simulink library "Lib_EMTAT"  (R2021b)
settings: Solver=VariableStepAuto  StartTime=0.0  StopTime=10.0  RelTol=1e-3
undefined symbols (not defined in the file or in its folder): A_M, B_M, Cj, component_degradation_input, Cs, E0_M, f_sw, K_M, MWS, Q_M, Q_rr, r_c, r_D, R_M, Rj, Ru, SNR_DX_M, SNR_IC_M, SNR_Mn_M, SNR_Mx_M, SOC_Init_M, u_ce0, u_D0
libraries: $bdroot x82, simulink x23, Lib_Dyn_StateSpace_EMTAT x3, PB_Library_Master_Working x1
(part 7 of 7)

== system Lib_EMTAT/Components/Power Flow/Three Phase Electric Machine (Source)/Open Circuit Failure - Line-Neutral Voltage ==
  Failed? : Inport
  V_LN_rms : Inport  Port=2
  Constant : Constant  Value=0
  IsInf : RelationalOperator  Operator=isInf  OutDataTypeStr=boolean  RndMeth=Simplest
  IsNaN : RelationalOperator  Operator=isNaN  OutDataTypeStr=boolean  RndMeth=Simplest
  Logical Operator : Logic  Operator=OR  Inputs=3  AllPortsSameDT=off  OutDataTypeStr=boolean
  Switch : Switch  Criteria=u2 > Threshold
  "V_LN_rms " : Outport
  wires:
  IsInf/1 -> Logical Operator/3
  IsNaN/1 -> Logical Operator/2
  Logical Operator/1 -> Switch/2
  Switch/1 -> "V_LN_rms "/1
  V_LN_rms/1 -> Switch/3, IsInf/1, IsNaN/1
  Constant/1 -> Switch/1
  Failed?/1 -> Logical Operator/1

== system Lib_EMTAT/Components/Power Flow/Three Phase Electric Machine (Source)/Open Circuit// Degradation Failure ==
  Eff : Inport
  DegFail? : Inport  Port=2
  OCFail? : Inport  Port=3
  Deg : Inport  Port=4
  Constant : Constant  Value=0
  Constant1 : Constant
  Divide : Product  Inputs=**
  "If degradation failure, penalize Eff." : Switch  Criteria=u2 > Threshold
  "If open circuit failure, set Eff = 0." : Switch  Criteria=u2 > Threshold
  Sum : Sum  Inputs=+-|
  "Eff " : Outport
  wires:
  Sum/1 -> Divide/1
  Constant1/1 -> Sum/1
  Constant/1 -> "If open circuit failure, set Eff = 0."/1
  OCFail?/1 -> "If open circuit failure, set Eff = 0."/2
  "If open circuit failure, set Eff = 0."/1 -> "Eff "/1
  Deg/1 -> Sum/2
  Divide/1 -> "If degradation failure, penalize Eff."/1
  Eff/1 -> "If degradation failure, penalize Eff."/3, Divide/2
  "If degradation failure, penalize Eff."/1 -> "If open circuit failure, set Eff = 0."/3
  DegFail?/1 -> "If degradation failure, penalize Eff."/2

== system Lib_EMTAT/Numerical Methods/Newton Raphson Solver/NR Update/Bounding ==
  note: Throw warning if solver independents reach independent limits.
  note: Throw error if initial condition is zero. This will disrupt normalization within solver.
  note: Throw error if initial conditions set in mask are not within independent limits set in mask.
  x(n+1)raw : Inport
  HitLimits : Subsystem
  ICsOutsideLimit : Subsystem
  Initial Conditions : Constant  Value=NR_IC_M
  Logical Operator{,1..3} (4 alike) : Logic  Operator=OR  AllPortsSameDT=off  OutDataTypeStr=boolean
  Memory : Memory  InheritSampleTime=on
  Memory1 : Memory  InheritSampleTime=on
  MinMax : MinMax  Inputs=2
  MinMax1 : MinMax  Function=max  Inputs=2
  Relational Operator : RelationalOperator  Operator===  OutDataTypeStr=boolean  RndMeth=Nearest
  Relational Operator1 : RelationalOperator  Operator===  OutDataTypeStr=boolean  RndMeth=Nearest
  Relational Operator2 : RelationalOperator  OutDataTypeStr=boolean  RndMeth=Nearest
  Relational Operator3 : RelationalOperator  Operator=<=  OutDataTypeStr=boolean  RndMeth=Nearest
  Relational Operator4 : RelationalOperator  Operator=isNaN  OutDataTypeStr=boolean  RndMeth=Nearest
  ZeroIC : Subsystem
  xBottom : Constant  Value=NR_Mn_Lim_M
  xTop : Constant  Value=NR_Mx_Lim_M
  x(n+1)Lim : Outport
  wires:
  Relational Operator4/1 -> ZeroIC/Enable
  [BotLim] -> Relational Operator3/2
  Relational Operator2/1 -> Logical Operator2/1
  Memory1/1 -> Logical Operator3/2
  Relational Operator3/1 -> Logical Operator2/2
  Logical Operator2/1 -> Logical Operator3/1
  [TopLim] -> Relational Operator2/2
  Initial Conditions/1 -> Relational Operator3/1, Relational Operator2/1, Relational Operator4/1
  Logical Operator3/1 -> Memory1/1, ICsOutsideLimit/Enable
  Logical Operator1/1 -> Memory/1, HitLimits/Enable
  Memory/1 -> Logical Operator1/2
  [HitBtm] -> Logical Operator/2
  Logical Operator/1 -> Logical Operator1/1
  [HitTop] -> Logical Operator/1
  Relational Operator/1 -> [HitTop]
  Relational Operator1/1 -> [HitBtm]
  MinMax/1 -> x(n+1)Lim/1, Relational Operator/2, Relational Operator1/1
  MinMax1/1 -> MinMax/2
  xTop/1 -> MinMax/1, Relational Operator/1, [TopLim]
  x(n+1)raw/1 -> MinMax1/1
  xBottom/1 -> Relational Operator1/2, MinMax1/2, [BotLim]

== system Lib_EMTAT/Numerical Methods/Newton Raphson Solver/NR Update/MatrixMult ==
  f(x(n)) : Inport
  inv(f'(x(n))) : Inport  Port=2
  Product : Product  Multiplication=Matrix(*)  RndMeth=Zero
  DTS : Outport
  wires:
  inv(f'(x(n)))/1 -> Product/1
  f(x(n))/1 -> Product/2
  Product/1 -> DTS/1

== system Lib_EMTAT/Numerical Methods/Newton Raphson Solver/NR Update/dxLimit1 ==
  dx : Inport
  f(x(n)) : Inport  Port=2
  Abs1 : Abs
  Constant : Constant  Value=0.5
  Constant1 : Constant  Value=-1
  Memory : Memory  InheritSampleTime=on
  MinMax : MinMax  Inputs=2
  MinMax1 : MinMax  Function=max  Inputs=2
  Product1 : Product  Inputs=3  RndMeth=Zero
  Product2 : Product  RndMeth=Zero
  Sum : Sum  Inputs=|++
  Threshold : Constant  Value=NR_dx_Lim_M/100
  dx_limited : Outport
  wires:
  MinMax1/1 -> dx_limited/1
  Constant1/1 -> Product2/1
  Product2/1 -> MinMax1/1
  MinMax/1 -> MinMax1/2
  dx/1 -> MinMax/2
  Abs1/1 -> MinMax/1, Product2/2
  Product1/1 -> Abs1/1
  Threshold/1 -> Product1/1
  f(x(n))/1 -> Memory/1, Sum/2
  Constant/1 -> Product1/2
  Memory/1 -> Sum/1
  Sum/1 -> Product1/3

== system Lib_EMTAT/Solvers/Iterative NR Solver w JacobianCalc/NRwCond/Iteration Conditions ==
  f(x) : Inport
  Abs : Abs
  Constant1 : Constant  Value=Cond_Limits_M
  Constant2 : Constant  Value=0
  Relational Operator : RelationalOperator  Operator=>  OutDataTypeStr=boolean  RndMeth=Nearest
  Relational Operator1 : RelationalOperator  Operator=>  OutDataTypeStr=boolean  RndMeth=Nearest
  Sum of Elements : Sum  Inputs=+
  Condition : Outport
  wires:
  Relational Operator1/1 -> Condition/1
  Sum of Elements/1 -> Relational Operator1/1
  Constant2/1 -> Relational Operator1/2
  Relational Operator/1 -> Sum of Elements/1
  f(x)/1 -> Abs/1
  Constant1/1 -> Relational Operator/2
  Abs/1 -> Relational Operator/1

== system Lib_EMTAT/Solvers/SS NR Solver w JacobianCalc /JacCalc w Reset/JC_Reset counter ==
  Reset Counter : Inport
  Count Condition : Inport  Port=2
  Constant1 : Constant  Value=SJacobianAttempts_M
  Data Type Conversion : DataTypeConversion
  Data Type Conversion1 : DataTypeConversion
  Logical Operator : Logic  Operator=NOT  AllPortsSameDT=off  OutDataTypeStr=boolean
  Product : Product  RndMeth=Zero
  Relational Operator : RelationalOperator  Operator===  OutDataTypeStr=boolean  RndMeth=Nearest
  Sum : Sum  Inputs=|++
  Unit Delay : UnitDelay  SampleTime=-1  HasFrameUpgradeWarning=on
  Unit Delay1 : UnitDelay  SampleTime=-1  HasFrameUpgradeWarning=on
  Unit Delay2 : UnitDelay  SampleTime=-1  HasFrameUpgradeWarning=on
  JC_Reset : Outport
  wires:
  Constant1/1 -> Relational Operator/1
  Relational Operator/1 -> JC_Reset/1
  Product/1 -> Sum/2
  Reset Counter/1 -> Unit Delay1/1
  Unit Delay/1 -> Product/2
  Data Type Conversion/1 -> Product/1
  Data Type Conversion1/1 -> Sum/1
  Unit Delay1/1 -> Logical Operator/1
  Logical Operator/1 -> Data Type Conversion/1
  Count Condition/1 -> Unit Delay2/1
  Unit Delay2/1 -> Data Type Conversion1/1
  Sum/1 -> Unit Delay/1, Relational Operator/2

== system Lib_EMTAT/Solvers/SS NR Solver w JacobianCalc /NewRaph w Cond/conditions ==
  f(x) : Inport
  Abs : Abs
  Constant2 : Constant  Value=Cond_Limits_M
  Constant3 : Constant  Value=0
  Relational Operator1 : RelationalOperator  Operator=>  OutDataTypeStr=boolean  RndMeth=Nearest
  Relational Operator2 : RelationalOperator  Operator=>  OutDataTypeStr=boolean  RndMeth=Nearest
  Sum of Elements : Sum  Inputs=+
  Condition : Outport
  wires:
  Constant2/1 -> Relational Operator1/2
  Relational Operator1/1 -> Sum of Elements/1
  Constant3/1 -> Relational Operator2/2
  Abs/1 -> Relational Operator1/1
  Sum of Elements/1 -> Relational Operator2/1
  f(x)/1 -> Abs/1
  Relational Operator2/1 -> Condition/1

== system Lib_EMTAT/Components/Physics-Based/Boost Converter/DC - DC Converter/ Dynamic State ==
  note: On Cycle
  note: Off Cycle
  note: the aDF must decrease L_M
  note: the aDF must decrease L_M
  x : Inport
  u : Inport  Port=2
  d : Inport  Port=3
  Action Port : ActionPort
  Constant : Constant
  Product{,1..3} (4 alike) : Product
  "State Space Model A1, B1, C1, D1" : Lib_Dyn_StateSpace_EMTAT/State Space Model  A_M=[0, 0; 0, -(Ron_M+RL_M)/L_M]  B_M=[0, -1/C_M; 1/L_M, 0]  C_M="[1,  0]"  D_M=[0, RC_M]
  "State Space Model A2, B2, C2, D2" : Subsystem  mask(State Space Model){A_M=[0, 1/C_M; -1/L_M, -(Ron_M+RC_M+RL_M)/L_M], B_M=[0, -1/C_M; 1/L_M, RC_M/L_M], C_M=[1,  RC_M], D_M=[0, -RC_M]}
      mask prompts: A_M "A_M - "A" Matrix"; B_M "B_M - "B" Matrix"; C_M "C_M - "C" Matrix"; D_M "D_M - "D" Matrix"
      mask help:
      | This block represents a state space model that can be placed within an interative subsytem (i.e. the Newton-Raphson solver).
      | The states, x, and inputs, u must be fed into the block. The outputs, y, and state derivatives, x_dot are computed
      | via the standard state space equations. Note that the integrator that computes the states by integrating
      | the state derivatives should be placed outside of the iterative subsystem so that multiple integration steps do not
      | occur per each timestep.
      |
      | Initial conditions must be specified in the integrator blocks, and ABCD matrices specified as block mask parameters.
      mask Display:
      | fprintf('x_dot = Ax+Bu\ny = Cx+Du')
      | port_label('input',1,'x')
      | port_label('input',2,'u')
      | port_label('output',1,'x_dot')
      | port_label('output',2,'y')
  Sum : Sum  Inputs=++|
  Sum1 : Sum  Inputs=++|
  Sum2 : Sum  Inputs=+-
  xdot : Outport  VectorParamsAs1DForOutWhenUnconnected=off
  VB : Outport  Port=2  VectorParamsAs1DForOutWhenUnconnected=off
  wires:
  "State Space Model A1, B1, C1, D1"/1 -> Product/1
  d/1 -> [d]
  Sum2/1 -> Product2/2, Product3/2
  Constant/1 -> Sum2/1
  [x] -> "State Space Model A1, B1, C1, D1"/1
  "State Space Model A1, B1, C1, D1"/2 -> Product1/1
  [u] -> "State Space Model A1, B1, C1, D1"/2
  [d] -> Product1/2, Product/2
  [d] -> Sum2/2
  u/1 -> [u]
  [x] -> "State Space Model A2, B2, C2, D2"/1(x)
  [u] -> "State Space Model A2, B2, C2, D2"/2(u)
  Product3/1 -> Sum1/2
  "State Space Model A2, B2, C2, D2"/2(y) -> Product3/1
  "State Space Model A2, B2, C2, D2"/1(x_dot) -> Product2/1
  Product2/1 -> Sum/2
  x/1 -> [x]
  Product1/1 -> Sum1/1
  Product/1 -> Sum/1
  Sum1/1 -> VB/1  "VB"
  Sum/1 -> xdot/1  "xdot"

== system Lib_EMTAT/Components/Physics-Based/Boost Converter/DC - DC Converter/Steady State ==
  note: the aDF must decrease L_M
  note: based on http://www.farnell.com/datasheets/2046154.pdf
  note: d
  note: y = C*x + D*u
  note: the aDF must decrease L_M
  note: the aDF must decrease L_M
  note: the aDF must decrease L_M
  u : Inport
  d : Inport  Port=2
  "T_Ambient " : Inport  Port=3
  Action Port : ActionPort
  Add{,1..3} (4 alike) : Sum
  Constant : Constant
  Constant1 : Constant  Value=[0, 0; 0, -(Ron_M+RL_M)/L_M]  VectorParams1D=off
  Constant2 : Constant  Value=[0, 1/C_M; -1/L_M, -(Ron_M+RC_M+RL_M)/L_M]  VectorParams1D=off
  Constant3 : Constant  Value=[0, -1/C_M; 1/L_M, RC_M/L_M]  VectorParams1D=off
  Constant4 : Constant  Value=[1, 0]  VectorParams1D=off
  Constant5 : Constant  Value=[0, RC_M]  VectorParams1D=off
  Constant6 : Constant  Value=[0, -1/C_M; 1/L_M, 0]  VectorParams1D=off
  Constant7 : Constant  Value=[1, RC_M]  VectorParams1D=off
  Constant8 : Constant  Value=[0, -RC_M]  VectorParams1D=off
  Display2 : Display
  Gain : Gain  Gain=-1
  "Heat Feedback " : Display
  Heat Feedback 1 : Display
  Matrix Divide : Product  Inputs=/  Multiplication=Matrix(*)
  "No Heat Feedback " : Display
  No Heat Feedback 1 : Display
  Product{,3..4,6..10} (8 alike) : Product
  Product1 : Product  Multiplication=Matrix(*)
  Product2 : Product  Multiplication=Matrix(*)
  Product5 : Product  Inputs=3  Multiplication=Matrix(*)
  Sum : Sum  Inputs=|+-
  Sum1 : Sum  Inputs=|++
  "TemperatureModifiedPerformanceTerm1 " : Subsystem
  "TemperatureModifiedPerformanceTerm2 " : Subsystem
  x : Outport  VectorParamsAs1DForOutWhenUnconnected=off
  VB : Outport  Port=2  VectorParamsAs1DForOutWhenUnconnected=off
  wires:
  Constant2/1 -> No Heat Feedback 1/1
  [TAmb] -> "TemperatureModifiedPerformanceTerm2 "/1(In1)
  [TAmb] -> "TemperatureModifiedPerformanceTerm1 "/1(In1)
  "T_Ambient "/1 -> [TAmb]
  "TemperatureModifiedPerformanceTerm2 "/1(Out1) -> Heat Feedback 1/1, Product3/1
  "TemperatureModifiedPerformanceTerm1 "/1(Out1) -> Product/1, "Heat Feedback "/1
  [d] -> Product/2
  [MatrixLook] -> "No Heat Feedback "/1
  Constant8/1 -> Product10/1
  Product6/1 -> Add1/2
  Add/1 -> Matrix Divide/1
  Constant7/1 -> Product8/1
  [d] -> Product7/2
  Add1/1 -> Product5/2
  Product8/1 -> Add2/2
  Product10/1 -> Add3/2
  Constant5/1 -> Product9/1
  [d] -> Sum/2
  Product1/1 -> Sum1/2
  Product5/1 -> Gain/1
  Sum/1 -> Product10/2, Product8/2, Product6/2, Product3/2
  Add3/1 -> Product1/1
  Constant/1 -> Sum/1
  Constant6/1 -> Product4/1
  [u] -> Product5/3
  [d] -> Product4/2
  Gain/1 -> x/1, Display2/1, Product2/2  "x"
  Constant4/1 -> Product7/1
  u/1 -> [u]
  Product2/1 -> Sum1/1
  d/1 -> [d]
  Product7/1 -> Add2/1
  Sum1/1 -> VB/1  "VB"
  Constant1/1 -> [MatrixLook]
  Product4/1 -> Add1/1
  [d] -> Product9/2
  Product/1 -> Add/1
  Constant3/1 -> Product6/1
  Product3/1 -> Add/2
  Matrix Divide/1 -> Product5/1
  Product9/1 -> Add3/1
  Add2/1 -> Product2/1
  [u] -> Product1/2

== system Lib_EMTAT/Components/Physics-Based/Boost Converter/Power Loss /VGateTempModified ==
  note: normalized to 25°C
  VGate : Inport
  TAmb : Inport  Port=2
  Add1 : Sum
  Constant7 : Constant  Value=25
  Multiply1 : Product
  Subtract : Sum  Inputs=+-
  "V DS temp coefficient " : Constant  Value=.64
  VGateMod : Outport  VectorParamsAs1DForOutWhenUnconnected=off
  wires:
  Add1/1 -> VGateMod/1
  "V DS temp coefficient "/1 -> Multiply1/2
  Subtract/1 -> Multiply1/1
  TAmb/1 -> Subtract/1
  VGate/1 -> Add1/1
  Constant7/1 -> Subtract/2
  Multiply1/1 -> Add1/2

== system Lib_EMTAT/Components/Physics-Based/Buck Converter/DC - DC Converter/ Dynamic State ==
  x : Inport
  u : Inport  Port=2
  d : Inport  Port=3
  Action Port : ActionPort
  Constant : Constant
  Product{,1..3} (4 alike) : Product
  "State Space Model A1, B1, C1, D1" : Lib_Dyn_StateSpace_EMTAT/State Space Model  A_M=[0, 1/C_M; -1/L_M, -(Ron_M+RC_M+RL_M)/L_M]  B_M=[0, -1/C_M; 1/L_M, RC_M/L_M]  C_M="[1,  RC_M]"  D_M=[0, -RC_M]
  "State Space Model A2, B2, C2, D2" : Lib_Dyn_StateSpace_EMTAT/State Space Model  A_M=[0, 1/C_M; -1/L_M, -(Ron_M+RC_M+RL_M)/L_M]  B_M=[0, -1/C_M; 0, RC_M/L_M]  C_M="[1,  RC_M]"  D_M=[0, -RC_M]
  Sum : Sum  Inputs=++|
  Sum1 : Sum  Inputs=++|
  Sum2 : Sum  Inputs=+-
  xdot : Outport  VectorParamsAs1DForOutWhenUnconnected=off
  VB : Outport  Port=2  VectorParamsAs1DForOutWhenUnconnected=off
  wires:
  Sum/1 -> xdot/1  "xdot"
  Sum1/1 -> VB/1  "VB"
  Product/1 -> Sum/1
  Product1/1 -> Sum1/1
  x/1 -> [x]
  Product2/1 -> Sum/2
  "State Space Model A2, B2, C2, D2"/1 -> Product2/1
  "State Space Model A2, B2, C2, D2"/2 -> Product3/1
  Product3/1 -> Sum1/2
  [u] -> "State Space Model A2, B2, C2, D2"/2
  [x] -> "State Space Model A2, B2, C2, D2"/1
  u/1 -> [u]
  [d] -> Sum2/2
  [d] -> Product/2, Product1/2
  [u] -> "State Space Model A1, B1, C1, D1"/2
  "State Space Model A1, B1, C1, D1"/2 -> Product1/1
  [x] -> "State Space Model A1, B1, C1, D1"/1
  Constant/1 -> Sum2/1
  Sum2/1 -> Product3/2, Product2/2
  d/1 -> [d]
  "State Space Model A1, B1, C1, D1"/1 -> Product/1

== system Lib_EMTAT/Components/Physics-Based/Buck Converter/DC - DC Converter/Steady State ==
  note: y = C*x + D*u
  note: d
  u : Inport
  d : Inport  Port=2
  "T_Ambient " : Inport  Port=3
  Action Port : ActionPort
  Add{,1..3} (4 alike) : Sum
  Constant : Constant
  Constant3 : Constant  Value=[0, -1/C_M; 0, RC_M/L_M]  VectorParams1D=off
  Constant4 : Constant  Value=[1, RC_M]  VectorParams1D=off
  Constant5 : Constant  Value=[0, -RC_M]  VectorParams1D=off
  Constant6 : Constant  Value=[0, -1/C_M; 1/L_M, RC_M]  VectorParams1D=off
  Constant7 : Constant  Value=[1, RC_M]  VectorParams1D=off
  Constant8 : Constant  Value=[0, -RC_M]  VectorParams1D=off
  Gain : Gain  Gain=-1
  Matrix Divide : Product  Inputs=/  Multiplication=Matrix(*)
  Product{,3..4,6..10} (8 alike) : Product
  Product1 : Product  Multiplication=Matrix(*)
  Product2 : Product  Multiplication=Matrix(*)
  Product5 : Product  Inputs=3  Multiplication=Matrix(*)
  Sum : Sum  Inputs=|+-
  Sum1 : Sum  Inputs=|++
  "TemperatureModifiedPerformanceTerm2 " : Subsystem
  x : Outport  VectorParamsAs1DForOutWhenUnconnected=off
  VB : Outport  Port=2  VectorParamsAs1DForOutWhenUnconnected=off
  wires:
  [u] -> Product1/2
  Add2/1 -> Product2/1
  Product9/1 -> Add3/1
  Matrix Divide/1 -> Product5/1
  Product3/1 -> Add/2
  Constant3/1 -> Product6/1
  Product/1 -> Add/1
  [d] -> Product9/2
  Product4/1 -> Add1/1
  Sum1/1 -> VB/1  "VB"
  Product7/1 -> Add2/1
  d/1 -> [d]
  Product2/1 -> Sum1/1
  u/1 -> [u]
  Constant4/1 -> Product7/1
  Gain/1 -> Product2/2, x/1  "x"
  [d] -> Product4/2
  [u] -> Product5/3
  Constant6/1 -> Product4/1
  Constant/1 -> Sum/1
  Add3/1 -> Product1/1
  Sum/1 -> Product3/2, Product6/2, Product8/2, Product10/2
  Product5/1 -> Gain/1
  Product1/1 -> Sum1/2
  [d] -> Sum/2
  Constant5/1 -> Product9/1
  [d] -> Product/2
  Product10/1 -> Add3/2
  Product8/1 -> Add2/2
  Add1/1 -> Product5/2
  [d] -> Product7/2
  Constant7/1 -> Product8/1
  Add/1 -> Matrix Divide/1
  Product6/1 -> Add1/2
  Constant8/1 -> Product10/1
  "TemperatureModifiedPerformanceTerm2 "/1(Out1) -> Product/1, Product3/1
  "T_Ambient "/1 -> "TemperatureModifiedPerformanceTerm2 "/1(TAmbient)

== system Lib_EMTAT/Components/Physics-Based/Buck Converter/Power Loss /VGateTempModified ==
  note: normalized to 25°C
  "VGate " : Inport
  TAmb : Inport  Port=2
  Add1 : Sum
  Constant7 : Constant  Value=25
  Multiply1 : Product
  Subtract : Sum  Inputs=+-
  "V DS temp coefficient " : Constant  Value=.64
  "VGateMod " : Outport  VectorParamsAs1DForOutWhenUnconnected=off
  wires:
  Multiply1/1 -> Add1/2
  Constant7/1 -> Subtract/2
  "VGate "/1 -> Add1/1
  TAmb/1 -> Subtract/1
  Subtract/1 -> Multiply1/1
  "V DS temp coefficient "/1 -> Multiply1/2
  Add1/1 -> "VGateMod "/1

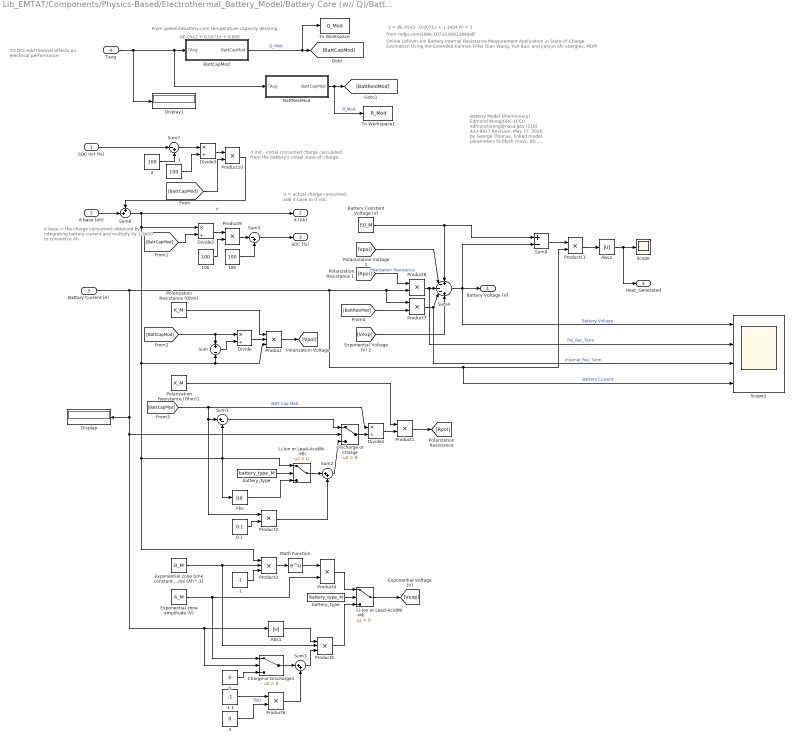
== system Lib_EMTAT/Components/Physics-Based/Electrothermal_Battery_Model/Battery Core (w// Q)/BatteryCore ==
  note: TO DO: Add thermal effects on electrical performance
  note: it = actual charge consumed.
      | add it base to it init.
  note: it init - initial consumed charge calculated
      | from the battery's initial state-of-charge.
  note: it base = the charge consumed;
      | obtained by integrating battery current
      | and multiply by 1/3600 to convert to Ah.
  note: Battery Model (Preliminary)
      | Edmond Wong/GRC-LCC0
      | edmond.wong@nasa.gov
      | (216) 433-8917
      |
      | Revision: May 17, 2018
      | by George Thomas, linked model
      | parameters to block mask, etc.
      |
      | Revision: April 29, 2019
      | by Mark Bell
      | Heat output, initial temperature feedback
  note: -9E-05x2 + 0.0071x + 0.868
  note: From greenlifebattery.com temperature-capacity derating
  note: y = 8E-05x2 - 0.0071x + 1.1424 R² = 1
  note: from mdpi.com/1996-1073/10/9/1284/pdf
  note: Online Lithium-Ion Battery Internal Resistance Measurement Application in State-of-Charge
      | Estimation Using the Extended Kalman Filter
      |
      | Dian Wang, Yun Bao, and Jianjun Shi
      |
      | energies, MDPI
  "SOC Init (%) " : Inport
  "it base (Ah) " : Inport  Port=2
  "Battery Current (A) " : Inport  Port=3
  "Tavg " : Inport  Port=4
  "-1 " : Constant  Value=-1
  -1 1 : Constant  Value=-1
  0 : Constant  Value=0
  0.1 : Constant  Value=0.1
  1 : Constant  Value=100
  100 : Constant  Value=100
  "100 " : Constant  Value=100
  2 : Constant  Value=100
  3 : Constant  Value=0
  Abs : Abs
  Abs1 : Abs
  Abs2 : Abs
  "BattCapMod " : Subsystem
  "BattResIMod " : Subsystem
  Battery Constant Voltage (V) : Constant  Value=E0_M
  Charge or Discharge1 : Switch  Criteria=u2 > Threshold
  Discharge or Charge : Switch  Criteria=u2 > Threshold
  Display : Display
  Display1 : Display
  Divide{,1..3} (4 alike) : Product  Inputs=*/
  Exponential zone amplitude (V) : Constant  Value=A_M
  Exponential zone time constant inverse (Ah^-1) : Constant  Value=B_M
  Li-Ion or Lead-Acid/Ni-Mh : Switch  Criteria=u2 > Threshold
  "Li-Ion or Lead-Acid/Ni-Mh " : Switch  Criteria=u2 > Threshold
  Math Function : Math  SignedPower=on  SaturateOnIntegerOverflow=on
  Polarization Resistance (Ohm) : Constant  Value=K_M
  Polarization Resistance (Ohm)1 : Constant  Value=K_M
  Product : Product  Inputs=3
  Product{1..2,4,6..11} (9 alike) : Product
  Product3 : Product  Inputs=3
  Product5 : Product  Inputs=3
  Scope : Scope
  Scope1 : Scope  NumInputPorts=4
  Sum : Sum  Inputs=+||-
  Sum1 : Sum  Inputs=|+-
  Sum2 : Sum  Inputs=|++
  Sum3 : Sum  Inputs=|++
  Sum4 : Sum  Inputs=+---+
  Sum5 : Sum  Inputs=|-+
  Sum6 : Sum  Inputs=++|
  Sum7 : Sum  Inputs=|-+
  Sum8 : Sum  Inputs=+-
  To Workspace : ToWorkspace  VariableName=Q_Mod  SampleTime=-1
  To Workspace1 : ToWorkspace  VariableName=R_Mod  SampleTime=-1
  battery_type : Constant  Value=battery_type_M
  "battery_type " : Constant  Value=battery_type_M
  Battery Voltage (V) : Outport  VectorParamsAs1DForOutWhenUnconnected=off
  it (Ah) : Outport  Port=2  VectorParamsAs1DForOutWhenUnconnected=off
  SOC (%) : Outport  Port=3  VectorParamsAs1DForOutWhenUnconnected=off
  Heat_Generated : Outport  Port=4  VectorParamsAs1DForOutWhenUnconnected=off
  wires:
  [BattResIMod] -> Product7/2
  "Tavg "/1 -> Display1/1, "BattCapMod "/1(TAvg), "BattResIMod "/1(TAvg)
  "BattResIMod "/1(BattCapMod) -> To Workspace1/1, [BattResIMod]  "R_Mod"
  [BattCapMod] -> Divide/1, Sum/1
  [BattCapMod] -> Divide2/2
  "BattCapMod "/1(BattCapMod) -> To Workspace/1, [BattCapMod]  "Q_Mod"
  "SOC Init (%) "/1 -> Sum7/1
  Product9/1 -> Sum5/1
  Divide3/1 -> Product10/1
  "100 "/1 -> Sum5/2
  2/1 -> Sum7/2
  Sum7/1 -> Divide3/1
  Product10/1 -> Sum6/1
  "it base (Ah) "/1 -> Sum6/2
  1/1 -> Divide3/2
  Polarization Resistance (Ohm)1/1 -> Product1/1
  Divide/1 -> Product/2
  Product5/1 -> "Li-Ion or Lead-Acid/Ni-Mh "/3
  Product/1 -> [Vpol]
  Sum/1 -> Divide/2
  Product7/1 -> Scope1/3, Sum4/4  "Internal_Res_Term"
  Exponential zone amplitude (V)/1 -> Product4/2, Charge or Discharge1/1
  3/1 -> Product6/2  "TBD"
  Product8/1 -> Scope1/2, Sum4/3  "Pol_Res_Term"
  battery_type/1 -> Li-Ion or Lead-Acid/Ni-Mh/2
  [Vexp] -> Sum4/5
  "battery_type "/1 -> "Li-Ion or Lead-Acid/Ni-Mh "/2
  Product6/1 -> Sum3/2
  Sum6/1 -> Divide2/1, Product/3, Sum/2, Li-Ion or Lead-Acid/Ni-Mh/1, Sum1/2, Abs/1, Product3/1, it (Ah)/1  "it"
  [BattCapMod] -> Divide1/1, Product2/1, Sum1/1  "Batt Cap Mod"
  100/1 -> Product9/2
  "-1 "/1 -> Product3/3
  Charge or Discharge1/1 -> Sum3/1
  Math Function/1 -> Product4/1
  Divide2/1 -> Product9/1
  -1 1/1 -> Product6/1
  [Rpol] -> Product8/1  "Polarization Resistance"
  Sum1/1 -> Discharge or Charge/1
  [Vpol] -> Sum4/2
  Product4/1 -> "Li-Ion or Lead-Acid/Ni-Mh "/1
  Sum5/1 -> SOC (%)/1
  "Li-Ion or Lead-Acid/Ni-Mh "/1 -> [Vexp]
  Polarization Resistance (Ohm)/1 -> Product/1
  Product2/1 -> Sum2/2
  Abs1/1 -> Product5/1
  Discharge or Charge/1 -> Divide1/2
  0/1 -> Charge or Discharge1/3
  Abs/1 -> Li-Ion or Lead-Acid/Ni-Mh/3
  Exponential zone time constant inverse (Ah^-1)/1 -> Product5/2, Product3/2
  Sum2/1 -> Discharge or Charge/3
  Product3/1 -> Math Function/1
  Li-Ion or Lead-Acid/Ni-Mh/1 -> Sum2/1
  Sum3/1 -> Product5/3
  0.1/1 -> Product2/2
  Product1/1 -> [Rpol]
  Divide1/1 -> Product1/2
  Abs2/1 -> Heat_Generated/1, Scope/1
  Sum8/1 -> Product11/1
  Product11/1 -> Abs2/1
  Battery Constant Voltage (V)/1 -> Sum8/1, Sum4/1
  "Battery Current (A) "/1 -> Scope1/4, Product11/2, Product7/1, Product8/2, Discharge or Charge/2, Charge or Discharge1/2, Abs1/1, Display/1  "Battery Current"
  Sum4/1 -> Sum8/2, Battery Voltage (V)/1, Scope1/1  "Battery Voltage"
  [BattCapMod] -> Product10/2

== system Lib_EMTAT/Components/Power Flow/AC-AC Transformer/Compensate for Divide By Zero/Fix Divide By Zero. ==
  V_LN_rms_1 : Inport
  P_AC_1 : Inport  Port=2
  Constant : Constant  Value=0
  Divide1 : Product  Inputs=/*
  Switch : Switch  Criteria=u2 > Threshold
  I_L_rms_1 : Outport
  wires:
  Switch/1 -> I_L_rms_1/1
  P_AC_1/1 -> Divide1/2
  V_LN_rms_1/1 -> Divide1/1, Switch/2
  Divide1/1 -> Switch/1
  Constant/1 -> Switch/3

== system Lib_EMTAT/Components/Power Flow/AC-AC Transformer/Efficiency/Fix Divide By Zero. ==
  abs(P_AC_2) : Inport
  abs(P_AC_1) : Inport  Port=2
  Constant : Constant  Value=inf
  Divide1 : Product  Inputs=/*
  Switch : Switch  Criteria=u2 ~= 0
  Eff : Outport
  wires:
  abs(P_AC_2)/1 -> Switch/2, Divide1/1
  abs(P_AC_1)/1 -> Divide1/2
  Switch/1 -> Eff/1
  Divide1/1 -> Switch/1
  Constant/1 -> Switch/3

== system Lib_EMTAT/Components/Power Flow/AC-AC Transformer/Efficiency/Fix Divide By Zero.1 ==
  abs(P_AC_1) : Inport
  abs(P_AC_2) : Inport  Port=2
  Constant : Constant  Value=inf
  Divide1 : Product  Inputs=/*
  Switch : Switch  Criteria=u2 ~= 0
  Eff : Outport
  wires:
  Switch/1 -> Eff/1
  abs(P_AC_1)/1 -> Switch/2, Divide1/1
  Divide1/1 -> Switch/1
  abs(P_AC_2)/1 -> Divide1/2
  Constant/1 -> Switch/3

== system Lib_EMTAT/Components/Power Flow/AC-DC Rectifier/Compensate for Divide By Zero./Fix Divide By Zero. ==
  V_LN_rms : Inport
  PEquivAC : Inport  Port=2
  Constant : Constant  Value=inf
  Divide1 : Product  Inputs=/*
  Switch : Switch  Criteria=u2 ~= 0
  I_L_rms : Outport
  wires:
  PEquivAC/1 -> Divide1/2
  Switch/1 -> I_L_rms/1
  V_LN_rms/1 -> Divide1/1, Switch/2
  Divide1/1 -> Switch/1
  Constant/1 -> Switch/3

== system Lib_EMTAT/Components/Power Flow/AC-DC Rectifier/Efficiency1/Fix Divide By Zero. ==
  abs(P_AC) : Inport
  abs(P_DC) : Inport  Port=2
  Constant : Constant  Value=inf
  Divide1 : Product  Inputs=/*
  Switch : Switch  Criteria=u2 ~= 0
  Eff : Outport
  wires:
  abs(P_AC)/1 -> Divide1/1, Switch/2
  abs(P_DC)/1 -> Divide1/2
  Switch/1 -> Eff/1
  Divide1/1 -> Switch/1
  Constant/1 -> Switch/3

== system Lib_EMTAT/Components/Power Flow/AC-DC Rectifier/Efficiency1/Fix Divide By Zero.1 ==
  abs(P_DC) : Inport
  abs(P_AC) : Inport  Port=2
  Constant : Constant  Value=inf
  Divide1 : Product  Inputs=/*
  Switch : Switch  Criteria=u2 ~= 0
  Eff : Outport
  wires:
  Switch/1 -> Eff/1
  abs(P_AC)/1 -> Divide1/2
  abs(P_DC)/1 -> Divide1/1, Switch/2
  Divide1/1 -> Switch/1
  Constant/1 -> Switch/3

== system Lib_EMTAT/Components/Power Flow/DC-AC Inverter/Compensate for Divide By Zero/Fix Divide By Zero. ==
  V_DC : Inport
  PEquivDC : Inport  Port=2
  Constant : Constant  Value=0
  Divide1 : Product  Inputs=/*
  Switch : Switch  Criteria=u2 > Threshold
  I_DC : Outport
  wires:
  V_DC/1 -> Divide1/1, Switch/2
  PEquivDC/1 -> Divide1/2
  Switch/1 -> I_DC/1
  Divide1/1 -> Switch/1
  Constant/1 -> Switch/3

== system Lib_EMTAT/Components/Power Flow/DC-DC Converter (Set Output Voltage)/Compensate for Divide By Zero/Fix Divide By Zero. ==
  Vin : Inport
  Pin : Inport  Port=2
  Constant : Constant  Value=0  SampleTime=-1
  Divide1 : Product  Inputs=/*
  Switch : Switch  Criteria=u2 ~= 0
  Iin : Outport
  wires:
  Vin/1 -> Switch/2, Divide1/1
  Pin/1 -> Divide1/2
  Switch/1 -> Iin/1
  Divide1/1 -> Switch/1
  Constant/1 -> Switch/3

== system Lib_EMTAT/Components/Power Flow/DC-DC Converter (Set Output Voltage)/Efficiency/Fix Divide By Zero. ==
  abs(Pout) : Inport
  abs(Pin) : Inport  Port=2
  Constant : Constant  Value=0
  Divide1 : Product  Inputs=/*
  Switch : Switch  Criteria=u2 ~= 0
  Eff : Outport
  wires:
  Switch/1 -> Eff/1
  abs(Pin)/1 -> Divide1/2
  abs(Pout)/1 -> Switch/2, Divide1/1
  Constant/1 -> Switch/3
  Divide1/1 -> Switch/1

== system Lib_EMTAT/Components/Power Flow/DC-DC Converter (Set Output Voltage)/Efficiency/Fix Divide By Zero.1 ==
  abs(Pin) : Inport
  abs(Pout) : Inport  Port=2
  Constant : Constant  Value=0
  Divide1 : Product  Inputs=/*
  Switch : Switch  Criteria=u2 ~= 0
  Eff : Outport
  wires:
  abs(Pin)/1 -> Switch/2, Divide1/1
  abs(Pout)/1 -> Divide1/2
  Switch/1 -> Eff/1
  Divide1/1 -> Switch/1
  Constant/1 -> Switch/3

== system Lib_EMTAT/Components/Power Flow/DC-DC Converter (Regulate Output Voltage)/Compensate for Divide By Zero/Fix Divide By Zero. ==
  Vin : Inport
  Pin : Inport  Port=2
  Constant : Constant  Value=0
  Divide1 : Product  Inputs=/*
  Switch : Switch  Criteria=u2 ~= 0
  Iin : Outport
  wires:
  Switch/1 -> Iin/1
  Pin/1 -> Divide1/2
  Vin/1 -> Switch/2, Divide1/1
  Divide1/1 -> Switch/1
  Constant/1 -> Switch/3

== system Lib_EMTAT/Components/Power Flow/DC-DC Converter (Regulate Output Voltage)/Efficiency/Fix Divide By Zero. ==
  abs(Pout) : Inport
  abs(Pin) : Inport  Port=2
  Constant : Constant  Value=0
  Divide1 : Product  Inputs=/*
  Switch : Switch  Criteria=u2 ~= 0
  Eff : Outport
  wires:
  abs(Pout)/1 -> Switch/2, Divide1/1
  abs(Pin)/1 -> Divide1/2
  Switch/1 -> Eff/1
  Divide1/1 -> Switch/1
  Constant/1 -> Switch/3

== system Lib_EMTAT/Components/Power Flow/DC-DC Converter (Regulate Output Voltage)/Efficiency/Fix Divide By Zero.1 ==
  abs(Pin) : Inport
  abs(Pout) : Inport  Port=2
  Constant : Constant  Value=0
  Divide1 : Product  Inputs=/*
  Switch : Switch  Criteria=u2 ~= 0
  Eff : Outport
  wires:
  abs(Pout)/1 -> Divide1/2
  abs(Pin)/1 -> Switch/2, Divide1/1
  Divide1/1 -> Switch/1
  Constant/1 -> Switch/3
  Switch/1 -> Eff/1

== system Lib_EMTAT/Components/Power Flow/Energy Storage Device/Warnings/SOC <= 0% ==
  Trigger : TriggerPort  VariantControl=(inherit)
  MATLAB Function : MATLAB Function  TreatAsAtomicUnit=on

== system Lib_EMTAT/Components/Power Flow/Energy Storage Device/Warnings/SOC > 100% ==
  Trigger : TriggerPort  VariantControl=(inherit)
  MATLAB Function : MATLAB Function  TreatAsAtomicUnit=on

== system Lib_EMTAT/Components/Power Flow/Three Phase Electric Machine (Sink)/Compensate for Divide By Zero/Fix Divide By Zero. ==
  V_LN_rms : Inport
  PEquivElect : Inport  Port=2
  Constant : Constant  Value=0
  Divide1 : Product  Inputs=/*
  Divide2 : Product  Inputs=**
  Switch : Switch  Criteria=u2 ~= 0
  I_L_rms : Outport
  wires:
  Switch/1 -> I_L_rms/1
  PEquivElect/1 -> Divide1/2
  Divide1/1 -> Switch/1
  V_LN_rms/1 -> Divide2/2, Switch/2, Divide1/1
  Constant/1 -> Divide2/1
  Divide2/1 -> Switch/3

== system Lib_EMTAT/Components/Power Flow/Three Phase Electric Machine (Source)/Compensate for Divide By Zero/Fix Divide By Zero. ==
  N : Inport
  PEquivMech : Inport  Port=2
  Constant : Constant  Value=0
  Divide : Product  Inputs=**
  Divide1 : Product  Inputs=/*
  Switch : Switch  Criteria=u2 ~= 0
  T : Outport
  wires:
  PEquivMech/1 -> Divide1/2
  Switch/1 -> T/1
  Divide1/1 -> Switch/1
  N/1 -> Switch/2, Divide1/1, Divide/2
  Constant/1 -> Divide/1
  Divide/1 -> Switch/3

== system Lib_EMTAT/Components/Power Flow/Three Phase Electric Machine (Source)/Direction Determination/Subsystem ==
  Pelec : Inport
  Eff : Inport  Port=2
  Constant : Constant  Value=0
  Divide : Product  Inputs=**
  Divide2 : Product  Inputs=*/
  Switch : Switch  Criteria=u2 ~= 0
  PEquivMech : Outport
  wires:
  Switch/1 -> PEquivMech/1
  Pelec/1 -> Divide2/1
  Divide2/1 -> Switch/1
  Eff/1 -> Divide2/2, Switch/2, Divide/2
  Divide/1 -> Switch/3
  Constant/1 -> Divide/1

== system Lib_EMTAT/Numerical Methods/Newton Raphson Solver/NR Update/Bounding/HitLimits ==
  Enable : EnablePort
  MATLAB Function : MATLAB Function  TreatAsAtomicUnit=on

== system Lib_EMTAT/Numerical Methods/Newton Raphson Solver/NR Update/Bounding/ICsOutsideLimit ==
  Enable : EnablePort
  MATLAB Function : MATLAB Function  TreatAsAtomicUnit=on

== system Lib_EMTAT/Numerical Methods/Newton Raphson Solver/NR Update/Bounding/ZeroIC ==
  Enable : EnablePort
  MATLAB Function : MATLAB Function  TreatAsAtomicUnit=on

== system Lib_EMTAT/Components/Physics-Based/Boost Converter/DC - DC Converter/ Dynamic State/State Space Model A2, B2, C2, D2 ==
  note: y = C*x + D*u
  note: x_dot = A*x + B*u
  x : Inport
  u : Inport  Port=2
  Constant : Constant  Value=A_M  VectorParams1D=off
  Constant1 : Constant  Value=B_M  VectorParams1D=off
  Constant2 : Constant  Value=C_M  VectorParams1D=off
  Constant3 : Constant  Value=D_M  VectorParams1D=off
  Display{,1..3} (4 alike) : Display
  Product{1..4} (4 alike) : Product  Multiplication=Matrix(*)
  Sum : Sum  Inputs=|++
  Sum1 : Sum  Inputs=|++
  x_dot : Outport  VectorParamsAs1DForOutWhenUnconnected=off
  y : Outport  Port=2  VectorParamsAs1DForOutWhenUnconnected=off
  wires:
  Sum/1 -> x_dot/1, Display2/1
  x/1 -> [x], Display/1
  Sum1/1 -> y/1, Display3/1
  u/1 -> [u], Display1/1
  Constant/1 -> Product4/1
  [x] -> Product4/2
  [u] -> Product3/2
  Constant1/1 -> Product3/1
  Product4/1 -> Sum/1
  Product3/1 -> Sum/2
  Product2/1 -> Sum1/1
  Constant3/1 -> Product1/1
  [x] -> Product2/2
  Product1/1 -> Sum1/2
  [u] -> Product1/2
  Constant2/1 -> Product2/1

== system Lib_EMTAT/Components/Physics-Based/Boost Converter/DC - DC Converter/Steady State/TemperatureModifiedPerformanceTerm1  ==
  note: update with gradual degredation term later
  In1 : Inport
  Add5 : Sum
  Constant : Constant
  Constant11 : Constant  Value=-(L_M)
  Constant13 : Constant  Value=0
  Divide1 : Product  Inputs=*/
  "InductorResistance " : Constant  Value=RL_M
  Matrix Concatenate3 : Concatenate  Mode=Multidimensional array
  Matrix Concatenate4 : Concatenate  Mode=Multidimensional array
  Matrix Concatenate5 : Concatenate  Mode=Multidimensional array  ConcatenateDimension=2
  Product : Product
  "TModifiedROn " : Subsystem
  Out1 : Outport  VectorParamsAs1DForOutWhenUnconnected=off
  wires:
  Matrix Concatenate5/1 -> Out1/1
  In1/1 -> "TModifiedROn "/1(In1)
  "InductorResistance "/1 -> Add5/1
  "TModifiedROn "/1(Out1) -> Add5/2
  Constant13/1 -> Matrix Concatenate4/1, Matrix Concatenate4/2, Matrix Concatenate3/1
  Matrix Concatenate4/1 -> Matrix Concatenate5/1
  Divide1/1 -> Matrix Concatenate3/2
  Matrix Concatenate3/1 -> Matrix Concatenate5/2
  Add5/1 -> Divide1/1
  Product/1 -> Divide1/2
  Constant11/1 -> Product/1
  Constant/1 -> Product/2

== system Lib_EMTAT/Components/Physics-Based/Boost Converter/DC - DC Converter/Steady State/TemperatureModifiedPerformanceTerm2  ==
  note: update with gradual degredation term later
  note: update with gradual degredation term later
  In1 : Inport
  Add5 : Sum  Inputs=+++
  CapacitorResistance : Constant  Value=RC_M
  Constant : Constant  Value=-1/L_M
  Constant1 : Constant  Value=1/C_M
  Constant11 : Constant  Value=-(L_M)
  Constant13 : Constant  Value=0
  Constant2 : Constant
  Constant3 : Constant
  Divide : Product  Inputs=*/
  Divide1 : Product  Inputs=*/
  "InductorResistance " : Constant  Value=RL_M
  Matrix Concatenate3 : Concatenate  Mode=Multidimensional array
  Matrix Concatenate4 : Concatenate  Mode=Multidimensional array
  Matrix Concatenate5 : Concatenate  Mode=Multidimensional array  ConcatenateDimension=2
  Product : Product
  "TModifiedROn " : Subsystem
  Out1 : Outport  VectorParamsAs1DForOutWhenUnconnected=off
  wires:
  Constant1/1 -> Matrix Concatenate3/1
  CapacitorResistance/1 -> Add5/3
  Matrix Concatenate5/1 -> Out1/1
  In1/1 -> "TModifiedROn "/1(In1)
  "InductorResistance "/1 -> Add5/1
  "TModifiedROn "/1(Out1) -> Add5/2
  Constant13/1 -> Matrix Concatenate4/1
  Matrix Concatenate4/1 -> Matrix Concatenate5/1
  Divide1/1 -> Matrix Concatenate3/2
  Matrix Concatenate3/1 -> Matrix Concatenate5/2
  Add5/1 -> Divide1/1
  Divide/1 -> Matrix Concatenate4/2
  Constant/1 -> Divide/1
  Constant2/1 -> Divide/2
  Product/1 -> Divide1/2
  Constant11/1 -> Product/1
  Constant3/1 -> Product/2

== system Lib_EMTAT/Components/Physics-Based/Buck Converter/DC - DC Converter/Steady State/TemperatureModifiedPerformanceTerm2  ==
  TAmbient : Inport
  Add5 : Sum  Inputs=+++
  CapacitorResistance : Constant  Value=RC_M
  Constant : Constant  Value=-1/L_M
  Constant1 : Constant  Value=1/C_M
  Constant11 : Constant  Value=-(L_M)
  Constant13 : Constant  Value=0
  Divide1 : Product  Inputs=*/
  "InductorResistance " : Constant  Value=RL_M
  Matrix Concatenate3 : Concatenate  Mode=Multidimensional array
  Matrix Concatenate4 : Concatenate  Mode=Multidimensional array
  Matrix Concatenate5 : Concatenate  Mode=Multidimensional array  ConcatenateDimension=2
  "TModifiedROn " : Subsystem
  Out1 : Outport  VectorParamsAs1DForOutWhenUnconnected=off
  wires:
  Constant11/1 -> Divide1/2
  Add5/1 -> Divide1/1
  Matrix Concatenate3/1 -> Matrix Concatenate5/2
  Divide1/1 -> Matrix Concatenate3/2
  Matrix Concatenate4/1 -> Matrix Concatenate5/1
  Constant13/1 -> Matrix Concatenate4/1
  "TModifiedROn "/1(Out1) -> Add5/2
  "InductorResistance "/1 -> Add5/1
  TAmbient/1 -> "TModifiedROn "/1(In1)
  Matrix Concatenate5/1 -> Out1/1
  CapacitorResistance/1 -> Add5/3
  Constant1/1 -> Matrix Concatenate3/1
  Constant/1 -> Matrix Concatenate4/2

== system Lib_EMTAT/Components/Physics-Based/Electrothermal_Battery_Model/Battery Core (w// Q)/BatteryCore/BattCapMod  ==
  TAvg : Inport
  "A " : Constant  Value=-9e-05
  Add : Sum  Inputs=+++
  "B " : Constant  Value=0.0071
  Battery Capacity (Ah) : Constant  Value=Q_M
  C : Constant  Value=.868
  Constant : Constant
  Degradation Parameter Multiplier : $bdroot/Components/Physics-Based/Degradation Parameter Multiplier  SystemSampleTime=-1  VariantActivationTime=update diagram  Latency=0  AutoFrameSizeCalculation=off
  Multiply{,1..3} (4 alike) : Product
  Square : Math  Operator=square  SignedPower=on  SaturateOnIntegerOverflow=on
  BattCapMod : Outport  VectorParamsAs1DForOutWhenUnconnected=off
  wires:
  Multiply2/1 -> BattCapMod/1
  C/1 -> Add/3
  Multiply1/1 -> Add/2
  Add/1 -> Multiply2/2
  "A "/1 -> Multiply/2
  Multiply/1 -> Add/1
  Square/1 -> Multiply/1
  TAvg/1 -> Square/1, Multiply1/1
  "B "/1 -> Multiply1/2
  Constant/1 -> Degradation Parameter Multiplier/1
  Battery Capacity (Ah)/1 -> Multiply3/2
  Degradation Parameter Multiplier/1 -> Multiply3/1
  Multiply3/1 -> Multiply2/1

== system Lib_EMTAT/Components/Physics-Based/Electrothermal_Battery_Model/Battery Core (w// Q)/BatteryCore/BattResIMod  ==
  TAvg : Inport
  "A " : Constant  Value=8e-05
  Add : Sum  Inputs=+++
  "B " : Constant  Value=0.0071
  C : Constant  Value=1.1424
  Constant : Constant  Commented=on
  Degradation Parameter Multiplier : PB_Library_Master_Working/Degradation Parameter Multiplier  Commented=on  SystemSampleTime=-1  VariantActivationTime=update diagram  Latency=0  AutoFrameSizeCalculation=off
  Divide : Product  Commented=on  Inputs=/*
  Internal Resistance (Ohm) : Constant  Value=R_M
  Multiply : Product
  Multiply1 : Product
  Multiply2 : Product  Inputs=3
  Square : Math  Operator=square  SignedPower=on  SaturateOnIntegerOverflow=on
  BattCapMod : Outport  VectorParamsAs1DForOutWhenUnconnected=off
  wires:
  Multiply2/1 -> BattCapMod/1
  C/1 -> Add/3
  Multiply1/1 -> Add/2
  Add/1 -> Multiply2/3
  "A "/1 -> Multiply/2
  Multiply/1 -> Add/1
  Square/1 -> Multiply/1
  TAvg/1 -> Square/1, Multiply1/1
  "B "/1 -> Multiply1/2
  Divide/1 -> Multiply2/2
  Degradation Parameter Multiplier/1 -> Divide/1
  Internal Resistance (Ohm)/1 -> Multiply2/1
  Constant/1 -> Degradation Parameter Multiplier/1

== system Lib_EMTAT/Components/Physics-Based/Boost Converter/DC - DC Converter/Steady State/TemperatureModifiedPerformanceTerm1 /TModifiedROn  ==
  In1 : Inport
  Add4 : Sum
  Constant10 : Constant  Value=50
  Constant9 : Constant  Value=25
  Divide : Product  Inputs=*/
  Multiply : Product
  "OnResistance " : Constant  Value=Ron_M
  Out1 : Outport  VectorParamsAs1DForOutWhenUnconnected=off
  wires:
  In1/1 -> Add4/1
  Constant10/1 -> Divide/2
  Add4/1 -> Divide/1
  Constant9/1 -> Add4/2
  Divide/1 -> Multiply/2
  Multiply/1 -> Out1/1
  "OnResistance "/1 -> Multiply/1

== system Lib_EMTAT/Components/Physics-Based/Boost Converter/DC - DC Converter/Steady State/TemperatureModifiedPerformanceTerm2 /TModifiedROn  ==
  In1 : Inport
  Add4 : Sum
  Constant10 : Constant  Value=50
  Constant9 : Constant  Value=25
  Divide : Product  Inputs=*/
  Multiply : Product
  "OnResistance " : Constant  Value=Ron_M
  Out1 : Outport  VectorParamsAs1DForOutWhenUnconnected=off
  wires:
  In1/1 -> Add4/1
  Constant10/1 -> Divide/2
  Add4/1 -> Divide/1
  Constant9/1 -> Add4/2
  Divide/1 -> Multiply/2
  Multiply/1 -> Out1/1
  "OnResistance "/1 -> Multiply/1

== system Lib_EMTAT/Components/Physics-Based/Buck Converter/DC - DC Converter/Steady State/TemperatureModifiedPerformanceTerm2 /TModifiedROn  ==
  In1 : Inport
  Add4 : Sum
  Constant10 : Constant  Value=50
  Constant9 : Constant  Value=25
  Divide : Product  Inputs=*/
  Multiply : Product
  "OnResistance " : Constant  Value=Ron_M
  Out1 : Outport  VectorParamsAs1DForOutWhenUnconnected=off
  wires:
  "OnResistance "/1 -> Multiply/1
  Multiply/1 -> Out1/1
  Divide/1 -> Multiply/2
  Constant9/1 -> Add4/2
  Add4/1 -> Divide/1
  Constant10/1 -> Divide/2
  In1/1 -> Add4/1

== matlab function Lib_EMTAT/Components/Power Flow/Current Distribution/MATLAB Function ==
  data: I input; Isplit output double; Idmd input
function Isplit = splitBranches1(I, Idmd)

yi = zeros(length(Idmd),1); %initialize vector in for loop.
if length(I) == length(Idmd)
    yi = I.*Idmd./sum(Idmd);
else
    for i = 1:1:length(I)

            yi(i*length(I)-length(I)+1:i*length(I),1) = I(i).*Idmd(i*length(I)-length(I)+1:i*length(I))./sum(Idmd(i*length(I)-length(I)+1: i*length(I)));
    end
end
Isplit = yi;

== matlab function Lib_EMTAT/Numerical Methods/Jacobian Calculator/Jacobian/Jacobian Calc ==
  data: IterationIn input; XpOut output; y_xpIn input; PerIn input; XoIn input; InvJOut output; JOut output; JStateIn input; y_StateIn input; y_StateOut output; Er input; ErSv output
function [XpOut, InvJOut, JOut, y_StateOut, ErSv] = fcn(IterationIn, y_xpIn, PerIn, XoIn, JStateIn, y_StateIn, Er)

% Set inital condiations
i = IterationIn;
XpOut = XoIn;
InvJOut = zeros(length(XoIn));
JOut = JStateIn;
y_StateOut = y_StateIn;
PerVec = reshape(PerIn',1,[]);
LenPV = length(PerVec);
LenXo = length(XoIn);
ErSv = Er;

% Begin taking data from f(x) at iteration a+1
a = 1;
% Begin determining Jacobian at iteration b+1
b = a+1;

% Set Xp Output
if i > a && i <= LenPV + a
    current_Xp = mod(i-a-1,LenXo)+1;
    XpOut(current_Xp) = XpOut(current_Xp) + PerVec(i - a);
end

% save state feedback
if LenXo == 1
    if i >= b;
        y_StateOut(i-a) = y_xpIn;
    end
else
    if i > a && i<= LenPV + a+1;
        y_StateOut(:,i - a) = y_xpIn;
    end
end

% Create Jacobian
if i == LenPV + b
    % Generate Jacobian matrices for each set, stacked.
    if LenXo == 1
        JMtx_extended = (y_StateOut(2:end)' - repmat(y_StateOut(1),1,LenPV))./PerVec;
    else
        JMtx_extended = (y_StateOut(:,2:end) - repmat(y_StateOut(:,1),1,LenPV))./repmat(PerVec,LenXo,1);
    end
    
    % Initialize sum matricies
    JMtrx_sum = zeros(LenXo);
    Nsum = zeros(LenXo);
    
    % determine how many perturbation sets there are, b/c MATLAB likes to
    % flip vectors when they enter MATLAB functions from Simulink for no reason.
    if min(size(PerIn)) == 1
     if LenXo == 1;
        PerNum = length(PerIn); 
     else 
        PerNum = 1;
     end
    else
        PerNum = size(PerIn,1);
    end
    
    for set = 1: PerNum
        % Break out Jacobian matrix for the current perturbation set
        JMtrx_cur = JMtx_extended(:, LenXo*(set-1)+1:LenXo*set);
        % Sum Jacobian matrices for each set
        JMtrx_sum = JMtrx_sum + JMtrx_cur(:,1:LenXo);
        % Sum number of acceptable values
        Nsum = Nsum + abs(sign(JMtrx_cur(:,1:LenXo)));
    end
    
    % Average Jacobian Matricies
    Javg = JMtrx_sum./max(Nsum,1);
    
    JOut = Javg;
    
    % Invert Jacobian
    if rank(JOut) == length(InvJOut)
        InvJOut = inv(JOut(:,:));
    elseif ErSv < 1
        disp('Jacobian can not be inverted.');
        ErSv = 1;
    end
end

== matlab function Lib_EMTAT/Components/Power Flow/Energy Storage Device/Warnings/SOC <= 0%/MATLAB Function ==
  data: BlkNm parameter
function fcn(BlkNm)
disp(['Warning in ' BlkNm ': State of charge is 0 percent.']);
end

== matlab function Lib_EMTAT/Components/Physics-Based/Buck Converter/DC - DC Converter/MATLAB Function ==
  data: A1 input; y output; dt input
function y  = switchLogic(A1, dt)    %A1 state martix, dt time step    

StableFlag=all(abs(1+dt*eig(A1))<=1);    %Forward Euler Stability requirement

if StableFlag==1
    y=1;    %runs dynamic model
    
else
    y=0;    %runs steady state model
    
end

end

== matlab function Lib_EMTAT/Components/Physics-Based/Boost Converter/DC - DC Converter/MATLAB Function ==
  data: A1 input; y output; dt input
function y  = switchLogic(A1, dt)    %A1 state martix, dt time step    

StableFlag=all(abs(1+dt*eig(A1))<=1);    %Forward Euler Stability requirement

if StableFlag==1
    y=1;    %runs dynamic model
    
else
    y=0;    %runs steady state model
    
end

end

== matlab function Lib_EMTAT/Components/Power Flow/Energy Storage Device/Warnings/SOC > 100%/MATLAB Function ==
  data: BlkNm parameter
function fcn(BlkNm)
disp(['Warning in ' BlkNm ': State of charge is greater than 100 percent.']);
end

== matlab function Lib_EMTAT/Numerical Methods/Newton Raphson Solver/NR Update/Bounding/HitLimits/MATLAB Function ==
  data: BlkNm_M parameter
function fcn(BlkNm_M)
%# Limit Newton Raphson outputs and produce a warning if it occurs
BName = BlkNm_M;
disp(['Warning in ' BName ': Solver limit has been hit, check for system convergence']);

== matlab function Lib_EMTAT/Numerical Methods/Newton Raphson Solver/NR Update/Bounding/ICsOutsideLimit/MATLAB Function ==
  data: BlkNm_M parameter
function ICNotInsideLimits(BlkNm_M)
%# Throw error if initial condition is outside bounds on independent.
BName = BlkNm_M;
error(['Error in ' BName ': Initial conditions, SNR_IC_M, of NR Solver are not within the Newton Raphson independent limits, SNR_Mx_M and SNR_Mn_M. Please choose initial condiitons conditions within the prescribed limits.']);

== matlab function Lib_EMTAT/Numerical Methods/Newton Raphson Solver/NR Update/Bounding/ZeroIC/MATLAB Function ==
  data: BlkNm_M parameter
function ICIsZero(BlkNm_M)
%# Throw error if initial condition is outside bounds on independent.
BName = BlkNm_M;
error(['Error in ' BName ': Initial conditions, SNR_IC_M, of NR Solver are zero. This will disrupt the normalization within the solver. Please choose non-zero numbers.']);

== matlab function Lib_EMTAT/Components/Power Flow/Electrical Bus/MATLAB Function ==
  data: u input; y output double; Nb parameter
function y = sumBranches(u,Nb)
if length(u)~=Nb
    yi = zeros(Nb,1); %initialize vector in for loop.
    for i = 1:1:length(u)/Nb
        yi(i) = sum(u(i:Nb:length(u)));
    end
else
    yi = sum(u);
end
y = yi;

== matlab function Lib_EMTAT/Components/Power Flow/Power Supply (Set Voltage)/MATLAB Function ==
  data: u input; y output double; Nb parameter
function y = sumBranches(u,Nb)
if length(u)~=Nb
    yi = zeros(Nb,1); %initialize vector in for loop.
    for i = 1:1:length(u)/Nb
        yi(i) = sum(u(i:Nb:length(u)));
    end
else
    yi = sum(u);
end
y = yi;

== matlab function Lib_EMTAT/Components/Power Flow/Current Junction/MATLAB Function ==
  data: u input; y output double; Nb parameter
function y = sumBranches(u,Nb)
yi = zeros(Nb,1); %initialize vector in for loop.
for i = 0:1:Nb-1
    if i ==0
        yi(i+1) = sum(u(1:Nb));
    end
    yi(i+1) = sum(u(i*Nb+1:i*Nb+Nb));
end
y = yi;
